simulink model "MSDRPrimaryLoop_LoadFollow"  (R2021b)
settings: Solver=VariableStepAuto  StartTime=0.0  StopTime=604900  MaxStep=1  MinStep=0.01  RelTol=1e-3
undefined symbols (not defined in the file): a_f, A_free_PHX, a_g, A_h_PHX, beta, beta_t, bubbleGeneratorArea, bubbleGeneratorDh, bubbleGeneratorElevation, bubbleGeneratorLength, bubbleGeneratorVolume, bubbleSaturationLevel, bubbleSeparatorArea, bubbleSeparatorDiameter, bubbleSeparatorDo, bubbleSeparatorLength, bubbleSeparatorSlope, bypassRatio, C0, coreFlowArea, coreFuelVolume, coreLowerPlenumArea, coreLowerPlenumHydraulicDiameter, coreLowerPlenumLength, coreLowerPlenumVolume, coreUpperPlenumArea, coreUpperPlenumHydraulicDiameter, coreUpperPlenumLength, coreUpperPlenumVolume, coreVolume, cpGraphite, dissolusionRatio, dMin, dScale, dsmConst, DXeG, Fiss_factor, fuelChannelHydrualicDiameter, fuelChannelLength, fuelDepositRatio, fuelFraction, fuelGraphiteArea, fuelGraphiteHeatTransferCoefficient, gamma0, gamma1, gamma2, generatorDsm, graphiteKDiff, graphiteUnitCellThickness, initialIodineConcentration, InitialXeMolarConcentration, InjectionRatio, injectionRatio, iodineDecayConstant, IodineDecayConstant, iodineYield, kGraphite, kScale, Lam, lam ... (+60)
libraries: fl_lib x268, nesl_utility x106, SimscapeFluids_lib x20, slpidlib x1
(part 3 of 12)

== system MSDRPrimaryLoop_LoadFollow/Pump/PumpPysical ==
  XeIn : Inport
  GasIn : Inport  Port=2
  Add : Sum  Inputs=|++
  Delay One Step : Delay  DelayLength=1
  Gain : Gain  Gain=0.5
  GasCalc : Subsystem
      settings: PortSchema="{\"entries\":[{\"content\":{\"sides\":[{\"content\":{\"connectorIds\":[\"In1\"]},\"type\":\"ConnectorPlacement.EquallySpacedRectSide\",\"uuid\":\"a8e1ce06-71c9-462d-8d5c-7a3e078b5544\"},{\"content\":{\"connectorIds\":[\"Out1\"],\"side\":\"RIGHT\"},\"type\":\"ConnectorPlacement.EquallySpacedRectSide\",\"uuid\":\"2c63a1ce-15e2-4b17-a432-f9f40781bd58\"},{\"content\":{\"connectorIds\":[\"LConn1\",\"LConn2\",\"LConn3\"],\"side\":\"TOP\"},\"type\":\"ConnectorPlacement.EquallySpacedRectSide\",\"uuid\":\"abc20e07-15eb-475f-be7f-cc96378523a1\"},{\"content\":{\"connectorIds\":[],\"side\":\"BOTTOM\"},\"type\":\"ConnectorPlacement.EquallySpacedRectSide\",\"uuid\":\"ab58f362-f4c2-4e86-bda0-802426066295\"}]},\"type\":\"ConnectorPlacement.EquallySpacedConnector\",\"uuid\":\"b54d49a9-048b-4912-bf18-92a7ef5e8aff\"}],\"packageUris\":[\"http://schema.mathworks.com/mf0/Connector/R2020b\"],\"version\":\"1.0\"}"
  PumpPhysics&Control : Subsystem
      settings: PortSchema="{\"entries\":[{\"content\":{\"sides\":[{\"content\":{\"connectorIds\":[\"LConn1\",\"In1\"]},\"type\":\"ConnectorPlacement.EquallySpacedRectSide\",\"uuid\":\"dfa2aa95-b0f6-4d42-b52c-ac64f68b4332\"},{\"content\":{\"connectorIds\":[\"RConn1\"],\"side\":\"RIGHT\"},\"type\":\"ConnectorPlacement.EquallySpacedRectSide\",\"uuid\":\"4e233f45-275b-4a62-b54f-a26261252d76\"},{\"content\":{\"connectorIds\":[],\"side\":\"TOP\"},\"type\":\"ConnectorPlacement.EquallySpacedRectSide\",\"uuid\":\"4d56cee6-54c9-4b53-b595-9dd9843d1812\"},{\"content\":{\"connectorIds\":[\"RConn2\"],\"side\":\"BOTTOM\"},\"type\":\"ConnectorPlacement.EquallySpacedRectSide\",\"uuid\":\"5b59abd0-5c01-4c9b-8b33-a5a665899d43\"}]},\"type\":\"ConnectorPlacement.EquallySpacedConnector\",\"uuid\":\"08118153-6206-4ac8-9187-5e3d4b128de1\"}],\"packageUris\":[\"http://schema.mathworks.com/mf0/Connector/R2020b\"],\"version\":\"1.0\"}"
  XenonCalc : Subsystem
      settings: PortSchema="{\"entries\":[{\"content\":{\"sides\":[{\"content\":{\"connectorIds\":[\"In1\"]},\"type\":\"ConnectorPlacement.EquallySpacedRectSide\",\"uuid\":\"2d0a178d-e3ce-4b60-98e7-1a8cc2d8e60a\"},{\"content\":{\"connectorIds\":[\"Out1\"],\"side\":\"RIGHT\"},\"type\":\"ConnectorPlacement.EquallySpacedRectSide\",\"uuid\":\"c836f1a2-1f60-4759-a54a-d13020949774\"},{\"content\":{\"connectorIds\":[\"LConn1\"],\"side\":\"TOP\"},\"type\":\"ConnectorPlacement.EquallySpacedRectSide\",\"uuid\":\"88d5b9ac-da0a-4ad3-844b-69cd646a8f29\"},{\"content\":{\"connectorIds\":[],\"side\":\"BOTTOM\"},\"type\":\"ConnectorPlacement.EquallySpacedRectSide\",\"uuid\":\"7af8c1ea-1928-402f-ba73-00fd41d484c9\"}]},\"type\":\"ConnectorPlacement.EquallySpacedConnector\",\"uuid\":\"10dc3dbd-7ee0-472f-a356-245132d02761\"}],\"packageUris\":[\"http://schema.mathworks.com/mf0/Connector/R2020b\"],\"version\":\"1.0\"}"
  Inlet : PMIOPort  Side=Left
  Outlet : PMIOPort  Port=2  Side=Right
  XeOut : Outport
  GasOut : Outport  Port=2
  wires:
  GasIn/1 -> GasCalc/1(GasIn), Add/1
  GasCalc/1(GasOut) -> GasOut/1, Add/2
  Add/1 -> Gain/1
  Gain/1 -> Delay One Step/1
  Delay One Step/1 -> PumpPhysics&Control/1(GasRef)
  XeIn/1 -> XenonCalc/1(XeIn)
  XenonCalc/1(XeOut) -> XeOut/1
  connections:
  Inlet/RConn1 -- GasCalc/LConn1 -- PumpPhysics&Control/LConn1
  Outlet/RConn1 -- PumpPhysics&Control/RConn1 -- GasCalc/LConn3
  PumpPhysics&Control/RConn2 -- GasCalc/LConn2 -- XenonCalc/LConn1

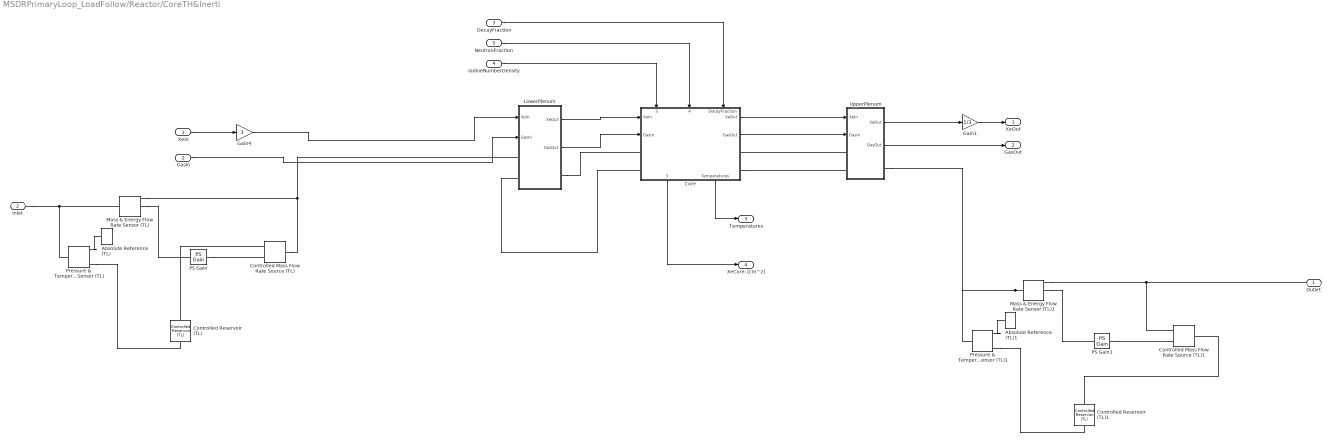
== system MSDRPrimaryLoop_LoadFollow/Reactor/CoreTH&Inerti ==
  XeIn : Inport
  GasIn : Inport  Port=2
  DecayFraction : Inport  Port=3
  IodineNumberDensity : Inport  Port=4
  NeutronFraction : Inport  Port=5
  Absolute Reference (TL) : fl_lib/Thermal Liquid/Elements/Absolute Reference (TL)
      settings: SourceProductBaseCode=SS
  Absolute Reference (TL)1 : fl_lib/Thermal Liquid/Elements/Absolute Reference (TL)
      settings: SourceProductBaseCode=SS
  Controlled Mass Flow Rate Source (TL) : fl_lib/Thermal Liquid/Sources/Controlled Mass Flow Rate Source (TL)  area=0.01 m^2
      settings: SourceProductBaseCode=SS  InternalSimscapePortConfiguration="{\"Bottom\":[],\"Left\":[{\"id\":\"A\",\"label\":\"A\",\"type\":\"foundation.thermal_liquid.thermal_liquid\"},{\"id\":\"M\",\"label\":\"M\",\"type\":\"input\"}],\"Right\":[{\"id\":\"B\",\"label\":\"B\",\"type\":\"foundation.thermal_liquid.thermal_liquid\"}],\"Top\":[]}"
  Controlled Mass Flow Rate Source (TL)1 : fl_lib/Thermal Liquid/Sources/Controlled Mass Flow Rate Source (TL)  area=0.01 m^2
      settings: SourceProductBaseCode=SS  InternalSimscapePortConfiguration="{\"Bottom\":[],\"Left\":[{\"id\":\"A\",\"label\":\"A\",\"type\":\"foundation.thermal_liquid.thermal_liquid\"},{\"id\":\"M\",\"label\":\"M\",\"type\":\"input\"}],\"Right\":[{\"id\":\"B\",\"label\":\"B\",\"type\":\"foundation.thermal_liquid.thermal_liquid\"}],\"Top\":[]}"
  Controlled Reservoir (TL) : fl_lib/Thermal Liquid/Elements/Controlled Reservoir (TL)  pressure_spec=foundation.enum.pressure_spec.atmospheric  reservoir_pressure=0.101325 MPa  area=0.01 m^2
      settings: SourceProductBaseCode=SS  InternalSimscapePortConfiguration="{\"Bottom\":[],\"Left\":[{\"id\":\"A\",\"label\":\"A\",\"type\":\"foundation.thermal_liquid.thermal_liquid\"}],\"Right\":[{\"id\":\"T_in\",\"label\":\"T\",\"type\":\"input\"}],\"Top\":[]}"
  Controlled Reservoir (TL)1 : fl_lib/Thermal Liquid/Elements/Controlled Reservoir (TL)  pressure_spec=foundation.enum.pressure_spec.atmospheric  reservoir_pressure=0.101325 MPa  area=0.01 m^2
      settings: SourceProductBaseCode=SS  InternalSimscapePortConfiguration="{\"Bottom\":[],\"Left\":[{\"id\":\"A\",\"label\":\"A\",\"type\":\"foundation.thermal_liquid.thermal_liquid\"}],\"Right\":[{\"id\":\"T_in\",\"label\":\"T\",\"type\":\"input\"}],\"Top\":[]}"
  Core : Subsystem
      settings: PortSchema="{\"entries\":[{\"content\":{\"sides\":[{\"content\":{\"connectorIds\":[\"In1\",\"In2\",\"LConn1\",\"LConn2\"]},\"type\":\"ConnectorPlacement.EquallySpacedRectSide\",\"uuid\":\"aa0e8e95-1a6b-4cbf-bd57-1ab05efc3e4b\"},{\"content\":{\"connectorIds\":[\"Out1\",\"Out2\",\"RConn1\",\"RConn2\"],\"side\":\"RIGHT\"},\"type\":\"ConnectorPlacement.EquallySpacedRectSide\",\"uuid\":\"e0eb6fcb-82a6-4aae-a4df-9b33aecd4e5c\"},{\"content\":{\"connectorIds\":[\"In3\",\"In4\",\"In5\"],\"side\":\"TOP\"},\"type\":\"ConnectorPlacement.EquallySpacedRectSide\",\"uuid\":\"5c074248-aee7-4f3a-b52e-673d2721cbd0\"},{\"content\":{\"connectorIds\":[\"Out3\",\"Out4\"],\"side\":\"BOTTOM\"},\"type\":\"ConnectorPlacement.EquallySpacedRectSide\",\"uuid\":\"89c6def1-6805-4ec7-892d-526461980e5e\"}]},\"type\":\"ConnectorPlacement.EquallySpacedConnector\",\"uuid\":\"cb503f6d-916e-44d8-aa57-58c36cce55e5\"}],\"packageUris\":[\"http://schema.mathworks.com/mf0/Connector/R2020b\"],\"version\":\"1.0\"}"
  Gain1 : Gain  Gain=1/3
  Gain4 : Gain  Gain=3
  LowerPlenum : Subsystem  mask{Volume=coreLowerPlenumVolume, Area=coreLowerPlenumArea, Length=coreLowerPlenumLength, Dh=coreLowerPlenumHydraulicDiameter, Elevation=coreLowerPlenumLength}
      mask prompts: Dh "Hydraulic Diameter"
  Mass & Energy Flow Rate Sensor (TL) : fl_lib/Thermal Liquid/Sensors/Mass & Energy Flow Rate Sensor (TL)
      settings: SourceProductBaseCode=SS  InternalSimscapePortConfiguration="{\"Bottom\":[],\"Left\":[{\"id\":\"A\",\"label\":\"A\",\"type\":\"foundation.thermal_liquid.thermal_liquid\"}],\"Right\":[{\"id\":\"B\",\"label\":\"B\",\"type\":\"foundation.thermal_liquid.thermal_liquid\"},{\"id\":\"M\",\"label\":\"M\",\"type\":\"output\"},{\"id\":\"PHI\",\"label\":\"Phi\",\"type\":\"output\"}],\"Top\":[]}"
  Mass & Energy Flow Rate Sensor (TL)1 : fl_lib/Thermal Liquid/Sensors/Mass & Energy Flow Rate Sensor (TL)
      settings: SourceProductBaseCode=SS  InternalSimscapePortConfiguration="{\"Bottom\":[],\"Left\":[{\"id\":\"A\",\"label\":\"A\",\"type\":\"foundation.thermal_liquid.thermal_liquid\"}],\"Right\":[{\"id\":\"B\",\"label\":\"B\",\"type\":\"foundation.thermal_liquid.thermal_liquid\"},{\"id\":\"M\",\"label\":\"M\",\"type\":\"output\"},{\"id\":\"PHI\",\"label\":\"Phi\",\"type\":\"output\"}],\"Top\":[]}"
  PS Gain : fl_lib/Physical Signals/Functions/PS Gain  gain=2
  PS Gain1 : fl_lib/Physical Signals/Functions/PS Gain  gain=2/3
  Pressure & Temperature Sensor (TL) : fl_lib/Thermal Liquid/Sensors/Pressure & Temperature Sensor (TL)
      settings: SourceProductBaseCode=SS  InternalSimscapePortConfiguration="{\"Bottom\":[],\"Left\":[{\"id\":\"A\",\"label\":\"A\",\"type\":\"foundation.thermal_liquid.thermal_liquid\"}],\"Right\":[{\"id\":\"B\",\"label\":\"B\",\"type\":\"foundation.thermal_liquid.thermal_liquid\"},{\"id\":\"P\",\"label\":\"P\",\"type\":\"output\"},{\"id\":\"T\",\"label\":\"T\",\"type\":\"output\"}],\"Top\":[]}"
  Pressure & Temperature Sensor (TL)1 : fl_lib/Thermal Liquid/Sensors/Pressure & Temperature Sensor (TL)
      settings: SourceProductBaseCode=SS  InternalSimscapePortConfiguration="{\"Bottom\":[],\"Left\":[{\"id\":\"A\",\"label\":\"A\",\"type\":\"foundation.thermal_liquid.thermal_liquid\"}],\"Right\":[{\"id\":\"B\",\"label\":\"B\",\"type\":\"foundation.thermal_liquid.thermal_liquid\"},{\"id\":\"P\",\"label\":\"P\",\"type\":\"output\"},{\"id\":\"T\",\"label\":\"T\",\"type\":\"output\"}],\"Top\":[]}"
  UpperPlenum : Subsystem  mask{Volume=coreUpperPlenumVolume, Area=coreUpperPlenumArea, Length=coreUpperPlenumLength, Dh=coreUpperPlenumHydraulicDiameter, Elevation=coreUpperPlenumLength}
      mask prompts: Dh "Hydraulic Diameter"
  Outlet : PMIOPort  Side=Right
  Inlet : PMIOPort  Port=2  Side=Left
  XeOut : Outport
  GasOut : Outport  Port=2
  Temperatures : Outport  Port=3
  "XeCore, [cm^2]" : Outport  Port=4
  wires:
  DecayFraction/1 -> Core/5(DecayFraction)
  NeutronFraction/1 -> Core/4(NeutronFraction)
  IodineNumberDensity/1 -> Core/3(IodineSNumberDensity)
  Core/3("TotalXeCrossSection, [cm^2]") -> "XeCore, [cm^2]"/1
  Core/4(Temperatures) -> Temperatures/1
  XeIn/1 -> Gain4/1
  Gain4/1 -> LowerPlenum/1(XeIn)
  GasIn/1 -> LowerPlenum/2(GasIn)
  LowerPlenum/1(XeOut) -> Core/1(XeIn)
  UpperPlenum/1(XeOut) -> Gain1/1
  Core/1(XeOut) -> UpperPlenum/1(XeIn)
  Core/2(GasOut) -> UpperPlenum/2(GasIn)
  LowerPlenum/2(GasOut) -> Core/2(GasIn)
  Gain1/1 -> XeOut/1
  UpperPlenum/2(GasOut) -> GasOut/1
  connections:
  LowerPlenum/LConn2 -- Core/LConn2
  Mass & Energy Flow Rate Sensor (TL)/RConn1 -- LowerPlenum/LConn1 -- Controlled Mass Flow Rate Source (TL)/RConn1
  LowerPlenum/RConn1 -- Core/LConn1
  UpperPlenum/LConn1 -- Core/RConn1
  Core/RConn2 -- UpperPlenum/LConn2
  Inlet/RConn1 -- Pressure & Temperature Sensor (TL)/LConn1 -- Mass & Energy Flow Rate Sensor (TL)/LConn1
  Pressure & Temperature Sensor (TL)/RConn1 -- Absolute Reference (TL)/LConn1
  Pressure & Temperature Sensor (TL)/RConn3 -- Controlled Reservoir (TL)/RConn1
  Controlled Reservoir (TL)/LConn1 -- Controlled Mass Flow Rate Source (TL)/LConn1
  Mass & Energy Flow Rate Sensor (TL)/RConn2 -- PS Gain/LConn1
  PS Gain/RConn1 -- Controlled Mass Flow Rate Source (TL)/LConn2
  Mass & Energy Flow Rate Sensor (TL)1/LConn1 -- UpperPlenum/RConn1 -- Pressure & Temperature Sensor (TL)1/LConn1
  Mass & Energy Flow Rate Sensor (TL)1/RConn1 -- Controlled Mass Flow Rate Source (TL)1/LConn1 -- Outlet/RConn1
  PS Gain1/RConn1 -- Controlled Mass Flow Rate Source (TL)1/LConn2
  Mass & Energy Flow Rate Sensor (TL)1/RConn2 -- PS Gain1/LConn1
  Pressure & Temperature Sensor (TL)1/RConn3 -- Controlled Reservoir (TL)1/RConn1
  Pressure & Temperature Sensor (TL)1/RConn1 -- Absolute Reference (TL)1/LConn1
  Controlled Reservoir (TL)1/LConn1 -- Controlled Mass Flow Rate Source (TL)1/RConn1

== system MSDRPrimaryLoop_LoadFollow/Reactor/Decay Heat ==
  note: Reference from UTK MSDR model
  (n/n_0) : Inport
  Decay Power Percentage : Fcn  Expr=u(2)+u(3)+u(4)
  Decay Precursor G1 : Fcn  Expr=u(1)*Fiss_factor*gamma0 - lambda0*u(2)
  Decay Precursor G2 : Fcn  Expr=u(1)*Fiss_factor*gamma1 - lambda1*u(3)
  Decay Precursor G3 : Fcn  Expr=u(1)*Fiss_factor*gamma2 - lambda2*u(4)
  Integrator : Integrator  InitialCondition=0.025125
  Integrator1 : Integrator  InitialCondition=0.0198578
  Integrator2 : Integrator  InitialCondition=0.0227606
  Mux : Mux
      settings: DisplayOption=signals
  "Relative Decay Power " : Outport  VectorParamsAs1DForOutWhenUnconnected=off
  wires:
  Decay Power Percentage/1 -> "Relative Decay Power "/1
  Decay Precursor G1/1 -> Integrator/1
  Decay Precursor G2/1 -> Integrator1/1
  Decay Precursor G3/1 -> Integrator2/1
  Mux/1 -> Decay Precursor G3/1, Decay Precursor G2/1, Decay Precursor G1/1, Decay Power Percentage/1
  Integrator/1 -> Mux/2
  Integrator1/1 -> Mux/3
  Integrator2/1 -> Mux/4
  (n/n_0)/1 -> Mux/1

== system MSDRPrimaryLoop_LoadFollow/Reactor/FlowFraction ==
  PS Abs : fl_lib/Physical Signals/Nonlinear Operators/PS Abs
      settings: SourceProductBaseCode=SS  InternalSimscapePortConfiguration="{\"Bottom\":[],\"Left\":[{\"id\":\"I\",\"label\":\"\",\"type\":\"input\"}],\"Right\":[{\"id\":\"O\",\"label\":\"\",\"type\":\"output\"}],\"Top\":[]}"
  PS Constant : fl_lib/Physical Signals/Sources/PS Constant  constant=nominalDischargeRate m^3/s
  PS Constant1 : fl_lib/Physical Signals/Sources/PS Constant  constant=0.1
  PS Divide : fl_lib/Physical Signals/Functions/PS Divide
      settings: SourceProductBaseCode=SS
  PS Max : fl_lib/Physical Signals/Nonlinear Operators/PS Max
      settings: SourceProductBaseCode=SS  InternalSimscapePortConfiguration="{\"Bottom\":[],\"Left\":[{\"id\":\"I1\",\"label\":\"\",\"type\":\"input\"},{\"id\":\"I2\",\"label\":\"\",\"type\":\"input\"}],\"Right\":[{\"id\":\"O\",\"label\":\"\",\"type\":\"output\"}],\"Top\":[]}"
  PS-Simulink Converter : nesl_utility/PS-Simulink Converter  PhysicalDomain=network_engine_domain  SubClassName=ps_output  LeftPortType=input  RightPortType=output  PseudoPeriodic=off  Frequencies=[]  Unit=inherit  AffineConversion=off
      settings: SourceProductBaseCode=PW,SS
  Volumetric Flow Rate Sensor (TL) : fl_lib/Thermal Liquid/Sensors/Volumetric Flow Rate Sensor (TL)
      settings: SourceProductBaseCode=SS  InternalSimscapePortConfiguration="{\"Bottom\":[],\"Left\":[{\"id\":\"A\",\"label\":\"A\",\"type\":\"foundation.thermal_liquid.thermal_liquid\"}],\"Right\":[{\"id\":\"B\",\"label\":\"B\",\"type\":\"foundation.thermal_liquid.thermal_liquid\"},{\"id\":\"V\",\"label\":\"V\",\"type\":\"output\"}],\"Top\":[]}"
  Outlet : PMIOPort  Side=Left
  Inlet : PMIOPort  Port=2  Side=Right
  FlowFrac : Outport
  wires:
  PS-Simulink Converter/1 -> FlowFrac/1
  connections:
  Inlet/RConn1 -- Volumetric Flow Rate Sensor (TL)/LConn1
  PS Divide/RConn1 -- PS Max/LConn1
  PS Abs/LConn1 -- Volumetric Flow Rate Sensor (TL)/RConn2
  PS Abs/RConn1 -- PS Divide/LConn1
  Volumetric Flow Rate Sensor (TL)/RConn1 -- Outlet/RConn1
  PS Constant/RConn1 -- PS Divide/LConn2
  PS Constant1/RConn1 -- PS Max/LConn2
  PS-Simulink Converter/LConn1 -- PS Max/RConn1

== system MSDRPrimaryLoop_LoadFollow/Reactor/Iodine ==
  NeutronFraction : Inport
  IodineAtoms : Integrator  InitialCondition=nominalFissionRate*iodineYield/iodineDecayConstant*initialIodineConcentration
  IodineDecay : Gain  Gain=iodineDecayConstant
  "IodineGeneration, [1/s]" : Product
  IodineYield : Constant  Value=iodineYield
  NominalFissionRate : Constant  Value=nominalFissionRate
  Product : Product
  Sum : Sum  Inputs=|+-
  TotalFuelMass : Gain  Gain=1/TotalFuelMass
  IodineSpecificNumberDensity : Outport
  wires:
  NeutronFraction/1 -> Product/1
  NominalFissionRate/1 -> Product/2
  Product/1 -> "IodineGeneration, [1/s]"/1
  IodineYield/1 -> "IodineGeneration, [1/s]"/2
  "IodineGeneration, [1/s]"/1 -> Sum/1
  Sum/1 -> IodineAtoms/1
  IodineAtoms/1 -> TotalFuelMass/1, IodineDecay/1
  IodineDecay/1 -> Sum/2
  TotalFuelMass/1 -> IodineSpecificNumberDensity/1

== system MSDRPrimaryLoop_LoadFollow/Reactor/Reactivity&PKE ==
  "XeCore, [cm^2]" : Inport
  FlowFrac : Inport  Port=2
  CORE TEMPERATURE : Inport  Port=3
  Ideal : Subsystem  Tag=Ideal  VariantControl=Ideal
      settings: PortSchema="{\"entries\":[{\"content\":{\"sides\":[{\"content\":{\"connectorIds\":[\"In1\",\"In2\"]},\"type\":\"ConnectorPlacement.EquallySpacedRectSide\",\"uuid\":\"074f11f6-c1de-4c2b-8a0d-6fb79ace2562\"},{\"content\":{\"connectorIds\":[\"Out1\"],\"side\":\"RIGHT\"},\"type\":\"ConnectorPlacement.EquallySpacedRectSide\",\"uuid\":\"1e53023e-28a9-4bb2-a66a-dc8b20408ca8\"},{\"content\":{\"connectorIds\":[\"In3\"],\"side\":\"TOP\"},\"type\":\"ConnectorPlacement.EquallySpacedRectSide\",\"uuid\":\"c85bb8ca-746f-4c14-b3fb-421abac5a8d5\"}]},\"type\":\"ConnectorPlacement.EquallySpacedConnector\",\"uuid\":\"7a35571e-b06b-4c7c-9209-bb340882391c\"}],\"packageUris\":[\"http://schema.mathworks.com/mf0/Connector/R2020b\"],\"version\":\"1.0\"}"
  Reactivity&PKE : Subsystem  Tag=PKE  VariantControl=PKE
      settings: PortSchema="{\"entries\":[{\"content\":{\"sides\":[{\"content\":{\"connectorIds\":[\"In1\",\"In2\"]},\"type\":\"ConnectorPlacement.EquallySpacedRectSide\",\"uuid\":\"074f11f6-c1de-4c2b-8a0d-6fb79ace2562\"},{\"content\":{\"connectorIds\":[\"Out1\"],\"side\":\"RIGHT\"},\"type\":\"ConnectorPlacement.EquallySpacedRectSide\",\"uuid\":\"1e53023e-28a9-4bb2-a66a-dc8b20408ca8\"},{\"content\":{\"connectorIds\":[],\"side\":\"TOP\"},\"type\":\"ConnectorPlacement.EquallySpacedRectSide\",\"uuid\":\"c85bb8ca-746f-4c14-b3fb-421abac5a8d5\"},{\"content\":{\"connectorIds\":[\"In3\"],\"side\":\"BOTTOM\"},\"type\":\"ConnectorPlacement.EquallySpacedRectSide\",\"uuid\":\"b54f140c-bd85-4d1d-bf3e-e1de5989b678\"}]},\"type\":\"ConnectorPlacement.EquallySpacedConnector\",\"uuid\":\"7a35571e-b06b-4c7c-9209-bb340882391c\"}],\"packageUris\":[\"http://schema.mathworks.com/mf0/Connector/R2020b\"],\"version\":\"1.0\"}"
  FRACTIONAL NEUTRON DENSITY : Outport

== system MSDRPrimaryLoop_LoadFollow/pipePHXToReactor/GasCalc ==
  GasIn : Inport
  Add : Sum  Inputs=+-
  GasExpansion : Subsystem  ReferencedSubsystem=GasExpansion
      settings: PortSchema="{\"entries\":[{\"content\":{\"sides\":[{\"content\":{\"connectorIds\":[\"LConn1\",\"In1\"]},\"type\":\"ConnectorPlacement.EquallySpacedRectSide\",\"uuid\":\"50c89675-cb8a-4964-af62-cb2014507b1d\"},{\"content\":{\"connectorIds\":[\"RConn1\",\"Out1\"],\"side\":\"RIGHT\"},\"type\":\"ConnectorPlacement.EquallySpacedRectSide\",\"uuid\":\"6b3adc78-0be5-4682-9da0-6fd41ffc4e71\"},{\"content\":{\"connectorIds\":[],\"side\":\"TOP\"},\"type\":\"ConnectorPlacement.EquallySpacedRectSide\",\"uuid\":\"5158b46f-a496-48e4-90d6-6c6dcc9e237b\"}]},\"type\":\"ConnectorPlacement.EquallySpacedConnector\",\"uuid\":\"7ff0188e-dc19-44a0-a8cf-bde33949414f\"}],\"packageUris\":[\"http://schema.mathworks.com/mf0/Connector/R2020b\"],\"version\":\"1.0\"}"
  Integrator : Integrator
  PS-Simulink Converter : nesl_utility/PS-Simulink Converter  PhysicalDomain=network_engine_domain  SubClassName=ps_output  LeftPortType=input  RightPortType=output  PseudoPeriodic=off  Frequencies=[]  Unit=inherit  AffineConversion=off
      settings: SourceProductBaseCode=PW,SS
  Product : Product
  VolumeToVoid : Gain  Gain=1/Volume
  Ref1 : PMIOPort  Side=Left
  VolumeRate : PMIOPort  Port=2  Side=Left
  Ref2 : PMIOPort  Port=3  Side=Left
  GasOut : Outport
  wires:
  VolumeToVoid/1 -> GasExpansion/1, Add/2
  Integrator/1 -> VolumeToVoid/1
  GasIn/1 -> Add/1
  Add/1 -> Product/1
  Product/1 -> Integrator/1
  PS-Simulink Converter/1 -> Product/2
  GasExpansion/1 -> GasOut/1
  connections:
  PS-Simulink Converter/LConn1 -- VolumeRate/RConn1
  GasExpansion/LConn1 -- Ref1/RConn1
  GasExpansion/RConn1 -- Ref2/RConn1

== system MSDRPrimaryLoop_LoadFollow/pipePHXToReactor/PLossFunc ==
  Constant : Constant  Value=Elevation*9.82
  PS-Simulink Converter : nesl_utility/PS-Simulink Converter  PhysicalDomain=network_engine_domain  SubClassName=ps_output  LeftPortType=input  RightPortType=output  PseudoPeriodic=off  Frequencies=[]  Unit=inherit  AffineConversion=off
      settings: SourceProductBaseCode=PW,SS
  PS-Simulink Converter1 : nesl_utility/PS-Simulink Converter  PhysicalDomain=network_engine_domain  SubClassName=ps_output  LeftPortType=input  RightPortType=output  PseudoPeriodic=off  Frequencies=[]  Unit=inherit  AffineConversion=off
      settings: SourceProductBaseCode=PW,SS
  Pressure & Temperature Sensor (TL) : fl_lib/Thermal Liquid/Sensors/Pressure & Temperature Sensor (TL)
      settings: SourceProductBaseCode=SS  InternalSimscapePortConfiguration="{\"Bottom\":[],\"Left\":[{\"id\":\"A\",\"label\":\"A\",\"type\":\"foundation.thermal_liquid.thermal_liquid\"}],\"Right\":[{\"id\":\"B\",\"label\":\"B\",\"type\":\"foundation.thermal_liquid.thermal_liquid\"},{\"id\":\"P\",\"label\":\"P\",\"type\":\"output\"},{\"id\":\"T\",\"label\":\"T\",\"type\":\"output\"}],\"Top\":[]}"
  Product : Product
  Subtract : Sum  Inputs=+-
  Thermodynamic Properties Sensor (TL) : fl_lib/Thermal Liquid/Sensors/Thermodynamic Properties Sensor (TL)
      settings: SourceProductBaseCode=SS  InternalSimscapePortConfiguration="{\"Bottom\":[],\"Left\":[{\"id\":\"A\",\"label\":\"A\",\"type\":\"foundation.thermal_liquid.thermal_liquid\"}],\"Right\":[{\"id\":\"U\",\"label\":\"u\",\"type\":\"output\"},{\"id\":\"RHO\",\"label\":\"rho\",\"type\":\"output\"},{\"id\":\"CP\",\"label\":\"cp\",\"type\":\"output\"}],\"Top\":[]}"
  Ref1 : PMIOPort  Side=Left
  Ref2 : PMIOPort  Port=2  Side=Right
  PLoss : Outport
  wires:
  PS-Simulink Converter1/1 -> Product/1
  PS-Simulink Converter/1 -> Subtract/1
  Product/1 -> Subtract/2
  Constant/1 -> Product/2
  Subtract/1 -> PLoss/1
  connections:
  Thermodynamic Properties Sensor (TL)/LConn1 -- Pressure & Temperature Sensor (TL)/RConn1 -- Ref2/RConn1
  PS-Simulink Converter/LConn1 -- Pressure & Temperature Sensor (TL)/RConn2
  Thermodynamic Properties Sensor (TL)/RConn2 -- PS-Simulink Converter1/LConn1
  Pressure & Temperature Sensor (TL)/LConn1 -- Ref1/RConn1

== system MSDRPrimaryLoop_LoadFollow/pipePHXToReactor/Subsystem ==
  note: Dh
  note: Dh
  note: Dh
  GasInRef : Inport
  2PModification : Subsystem  ReferencedSubsystem=TwoPhaseModification
      settings: PortSchema="{\"entries\":[{\"content\":{\"sides\":[{\"content\":{\"connectorIds\":[\"LConn1\"]},\"type\":\"ConnectorPlacement.EquallySpacedRectSide\",\"uuid\":\"7546b4b7-b669-49c8-8f27-f696391ea3ad\"},{\"content\":{\"connectorIds\":[\"RConn1\"],\"side\":\"RIGHT\"},\"type\":\"ConnectorPlacement.EquallySpacedRectSide\",\"uuid\":\"0e6176f2-177c-4327-bcfa-9a190fe9083f\"},{\"content\":{\"connectorIds\":[\"LConn2\"],\"side\":\"TOP\"},\"type\":\"ConnectorPlacement.EquallySpacedRectSide\",\"uuid\":\"16faf74c-4635-4009-a5b3-33dd03b625c6\"},{\"content\":{\"connectorIds\":[\"RConn2\",\"In1\"],\"side\":\"BOTTOM\"},\"type\":\"ConnectorPlacement.EquallySpacedRectSide\",\"uuid\":\"2081d73b-bb08-4ad9-b5c8-e48a4e9c4e20\"}]},\"type\":\"ConnectorPlacement.EquallySpacedConnector\",\"uuid\":\"243e4075-206b-4747-a8bc-b8f10d9a577f\"}],\"packageUris\":[\"http://schema.mathworks.com/mf0/Connector/R2020b\"],\"version\":\"1.0\"}"
  PS Abs : fl_lib/Physical Signals/Nonlinear Operators/PS Abs
      settings: SourceProductBaseCode=SS  InternalSimscapePortConfiguration="{\"Bottom\":[],\"Left\":[{\"id\":\"I\",\"label\":\"\",\"type\":\"input\"}],\"Right\":[{\"id\":\"O\",\"label\":\"\",\"type\":\"output\"}],\"Top\":[]}"
  Pipe (TL) : SimscapeFluids_lib/Thermal Liquid/Pipes & Fittings/Pipe (TL)  dynamic_compressibility=simscape.enum.onoff.on  inertia=simscape.enum.onoff.on  num_segments=1  pipe_length=Length m  area=Area m^2  Dh=0.1128 m  wall_spec=fluids.thermal_liquid.pipes_fittings.enum.wall_spec.rigid  Dh_rigid=Dh m  wall_compliance=1.2e-6 m/MPa  wall_time_constant=0.01 s  elevation_spec=foundation.enum.constant_variable.constant  elevation_gain=Elevation m  g=9.82 m/s^2  pressure_loss_spec=fluids.thermal_liquid.pipes_fittings.enum.PressureLossSpec.Haaland  length_add=1 m  roughness=15e-6 m  Re_friction_TLU=[400, 1000, 1500, 3000, 4000, 6000, 10000, 20000, 40000, 60000, 100000, 100000000]  friction_factor_TLU=[.264, .112, .071, .0417, .0387, .0268, .025, .0232, .0226, .022, .0214, .0214]  shape_factor=64  Re_lam=2000  Re_tur=4000  mdot_nominal=[.1, 1] kg/s  p_diff_nominal=[.001, .01] MPa  mdot_threshold=1e-6 kg/s  heat_transfer_spec=fluids.thermal_liquid.pipes_fittings.enum.HeatTransferSpec.Gnielinski  mdot_nominal_heat=[.1, 1] kg/s  T_in_nominal=[293.15, 293.15] K  T_out_nominal=[300, 300] K  p_in_nominal_heat=[.101325, .101325] MPa  T_wall_nominal=[303.15, 303.15] K  a_coeff=0.023  b_Re_power=0.8  c_Pr_power=0.4  Nu_lam=3.66  Re_Colburn_TLU=[100, 150, 1000]  Colburn_factor_TLU=[.019, .013, .002]  Re_Nu_TLU=[100, 150, 1000]  Pr_Nu_TLU=[1, 10]  Nu_TLU=[3.72, 4.21; 3.75, 4.44; 4.21, 7.15]  T0_vec=T0 K  p0_vec=P0 Pa  mdot0=0.1 kg/s
      settings: SourceProductBaseCode=SH  LogSimulationData=on
  Volumetric Flow Rate Sensor (TL) : fl_lib/Thermal Liquid/Sensors/Volumetric Flow Rate Sensor (TL)
      settings: SourceProductBaseCode=SS  InternalSimscapePortConfiguration="{\"Bottom\":[],\"Left\":[{\"id\":\"A\",\"label\":\"A\",\"type\":\"foundation.thermal_liquid.thermal_liquid\"}],\"Right\":[{\"id\":\"B\",\"label\":\"B\",\"type\":\"foundation.thermal_liquid.thermal_liquid\"},{\"id\":\"V\",\"label\":\"V\",\"type\":\"output\"}],\"Top\":[]}"
  Inlet : PMIOPort  Side=Left
  Outlet : PMIOPort  Port=2  Side=Right
  VolumeRate : PMIOPort  Port=3  Side=Right
  wires:
  GasInRef/1 -> 2PModification/1
  connections:
  Volumetric Flow Rate Sensor (TL)/RConn1 -- Pipe (TL)/LConn1
  Inlet/RConn1 -- 2PModification/LConn2 -- Volumetric Flow Rate Sensor (TL)/LConn1
  Pipe (TL)/RConn1 -- 2PModification/RConn2 -- 2PModification/LConn1
  Volumetric Flow Rate Sensor (TL)/RConn2 -- PS Abs/LConn1
  PS Abs/RConn1 -- VolumeRate/RConn1
  2PModification/RConn1 -- Outlet/RConn1

== system MSDRPrimaryLoop_LoadFollow/pipePHXToReactor/XenonCalc ==
  XeIn : Inport  OutDataTypeStr=double  Unit=kg/s
  PLoss : Inport  Port=2
  GasRef : Inport  Port=3
  Absolute Reference (TL) : fl_lib/Thermal Liquid/Elements/Absolute Reference (TL)
      settings: SourceProductBaseCode=SS
  Demux : Demux  Outputs=2
  Gas : Subsystem
      settings: PortSchema="{\"entries\":[{\"content\":{\"sides\":[{\"content\":{\"connectorIds\":[\"In1\"]},\"type\":\"ConnectorPlacement.EquallySpacedRectSide\",\"uuid\":\"9457d014-8c8c-4ede-953a-dad1b8fcff2e\"},{\"content\":{\"connectorIds\":[\"Out1\"],\"side\":\"RIGHT\"},\"type\":\"ConnectorPlacement.EquallySpacedRectSide\",\"uuid\":\"6b13e550-1648-4662-a58b-f6f49b8dfc45\"},{\"content\":{\"connectorIds\":[\"Out2\",\"In2\"],\"side\":\"TOP\"},\"type\":\"ConnectorPlacement.EquallySpacedRectSide\",\"uuid\":\"73a4211d-b4c2-4f72-9c26-6ee46c1777bd\"},{\"content\":{\"connectorIds\":[\"In3\",\"In4\"],\"side\":\"BOTTOM\"},\"type\":\"ConnectorPlacement.EquallySpacedRectSide\",\"uuid\":\"ca62b0cd-46c8-418f-9a8b-9558726bf444\"}]},\"type\":\"ConnectorPlacement.EquallySpacedConnector\",\"uuid\":\"020f2da1-56fe-4a8a-8a2d-2f75d9123e14\"}],\"packageUris\":[\"http://schema.mathworks.com/mf0/Connector/R2020b\"],\"version\":\"1.0\"}"
  InterphaseTranfser : Subsystem
      settings: PortSchema="{\"entries\":[{\"content\":{\"sides\":[{\"content\":{\"connectorIds\":[\"In1\",\"In2\",\"In3\"]},\"type\":\"ConnectorPlacement.EquallySpacedRectSide\",\"uuid\":\"d6303689-138e-451a-a3c3-60d601b4795c\"},{\"content\":{\"connectorIds\":[\"In5\",\"Out1\"],\"side\":\"RIGHT\"},\"type\":\"ConnectorPlacement.EquallySpacedRectSide\",\"uuid\":\"e99266db-1ad9-4248-a3a9-dc80edd4cbf2\"},{\"content\":{\"connectorIds\":[\"LConn1\"],\"side\":\"TOP\"},\"type\":\"ConnectorPlacement.EquallySpacedRectSide\",\"uuid\":\"07679a3e-e535-452f-8d16-cac9376cf8bb\"},{\"content\":{\"connectorIds\":[\"In4\"],\"side\":\"BOTTOM\"},\"type\":\"ConnectorPlacement.EquallySpacedRectSide\",\"uuid\":\"cd334689-6a33-4cbf-8721-40055306f60f\"}]},\"type\":\"ConnectorPlacement.EquallySpacedConnector\",\"uuid\":\"2a8870ca-366d-4312-85a0-e0a2095078d0\"}],\"packageUris\":[\"http://schema.mathworks.com/mf0/Connector/R2020b\"],\"version\":\"1.0\"}"
  Mux : Mux  Inputs=2
  PS Abs : fl_lib/Physical Signals/Nonlinear Operators/PS Abs
      settings: SourceProductBaseCode=SS  InternalSimscapePortConfiguration="{\"Bottom\":[],\"Left\":[{\"id\":\"I\",\"label\":\"\",\"type\":\"input\"}],\"Right\":[{\"id\":\"O\",\"label\":\"\",\"type\":\"output\"}],\"Top\":[]}"
  PS-Simulink Converter : nesl_utility/PS-Simulink Converter  PhysicalDomain=network_engine_domain  SubClassName=ps_output  LeftPortType=input  RightPortType=output  PseudoPeriodic=off  Frequencies=[]  Unit=inherit  AffineConversion=off
      settings: SourceProductBaseCode=PW,SS
  PS-Simulink Converter1 : nesl_utility/PS-Simulink Converter  PhysicalDomain=network_engine_domain  SubClassName=ps_output  LeftPortType=input  RightPortType=output  PseudoPeriodic=off  Frequencies=[]  Unit=inherit  AffineConversion=off
      settings: SourceProductBaseCode=PW,SS
  Pressure & Temperature Sensor (TL) : fl_lib/Thermal Liquid/Sensors/Pressure & Temperature Sensor (TL)
      settings: SourceProductBaseCode=SS  InternalSimscapePortConfiguration="{\"Bottom\":[],\"Left\":[{\"id\":\"A\",\"label\":\"A\",\"type\":\"foundation.thermal_liquid.thermal_liquid\"}],\"Right\":[{\"id\":\"B\",\"label\":\"B\",\"type\":\"foundation.thermal_liquid.thermal_liquid\"},{\"id\":\"P\",\"label\":\"P\",\"type\":\"output\"},{\"id\":\"T\",\"label\":\"T\",\"type\":\"output\"}],\"Top\":[]}"
  Salt : Subsystem
      settings: PortSchema="{\"entries\":[{\"content\":{\"sides\":[{\"content\":{\"connectorIds\":[\"In1\",\"In2\",\"In3\"]},\"type\":\"ConnectorPlacement.EquallySpacedRectSide\",\"uuid\":\"9457d014-8c8c-4ede-953a-dad1b8fcff2e\"},{\"content\":{\"connectorIds\":[\"Out1\"],\"side\":\"RIGHT\"},\"type\":\"ConnectorPlacement.EquallySpacedRectSide\",\"uuid\":\"6b13e550-1648-4662-a58b-f6f49b8dfc45\"},{\"content\":{\"connectorIds\":[\"In4\",\"In5\"],\"side\":\"TOP\"},\"type\":\"ConnectorPlacement.EquallySpacedRectSide\",\"uuid\":\"73a4211d-b4c2-4f72-9c26-6ee46c1777bd\"},{\"content\":{\"connectorIds\":[\"Out2\",\"In6\"],\"side\":\"BOTTOM\"},\"type\":\"ConnectorPlacement.EquallySpacedRectSide\",\"uuid\":\"ca62b0cd-46c8-418f-9a8b-9558726bf444\"}]},\"type\":\"ConnectorPlacement.EquallySpacedConnector\",\"uuid\":\"020f2da1-56fe-4a8a-8a2d-2f75d9123e14\"}],\"packageUris\":[\"http://schema.mathworks.com/mf0/Connector/R2020b\"],\"version\":\"1.0\"}"
  Volumetric Flow Rate Sensor (TL) : fl_lib/Thermal Liquid/Sensors/Volumetric Flow Rate Sensor (TL)
      settings: SourceProductBaseCode=SS  InternalSimscapePortConfiguration="{\"Bottom\":[],\"Left\":[{\"id\":\"A\",\"label\":\"A\",\"type\":\"foundation.thermal_liquid.thermal_liquid\"}],\"Right\":[{\"id\":\"B\",\"label\":\"B\",\"type\":\"foundation.thermal_liquid.thermal_liquid\"},{\"id\":\"V\",\"label\":\"V\",\"type\":\"output\"}],\"Top\":[]}"
  Inlet : PMIOPort  Side=Left
  Outlet : PMIOPort  Port=2  Side=Right
  XeOut : Outport
  wires:
  XeIn/1 -> Demux/1
  PS-Simulink Converter/1 -> InterphaseTranfser/5(VolumeRate), Gas/4(VolumeRate), Salt/5(VolumeRate)
  GasRef/1 -> Gas/3(GasRef), InterphaseTranfser/2(GasRef), Salt/4(GasRef)
  Demux/1 -> Salt/1(XeLIn)
  [IodineSNDensity] -> Salt/2(IodineSNumberDensity)
  Demux/2 -> Gas/1(XeGIn)
  Salt/1(XeLOut) -> Mux/1
  Gas/1(XeGOut) -> Mux/2
  Mux/1 -> XeOut/1
  Salt/2(GxSalt) -> InterphaseTranfser/1(GxSalt)
  Gas/2(GxGas) -> InterphaseTranfser/3(GxGas)
  InterphaseTranfser/1(TranfserRate) -> Salt/6(Interphase), Gas/2(Interphase)
  PS-Simulink Converter1/1 -> Salt/3(T_f_ave)
  PLoss/1 -> InterphaseTranfser/4(PLoss)
  connections:
  Outlet/RConn1 -- Volumetric Flow Rate Sensor (TL)/RConn1 -- InterphaseTranfser/LConn1
  Volumetric Flow Rate Sensor (TL)/LConn1 -- Pressure & Temperature Sensor (TL)/LConn1 -- Inlet/RConn1
  Volumetric Flow Rate Sensor (TL)/RConn2 -- PS Abs/LConn1
  PS Abs/RConn1 -- PS-Simulink Converter/LConn1
  Pressure & Temperature Sensor (TL)/RConn1 -- Absolute Reference (TL)/LConn1
  Pressure & Temperature Sensor (TL)/RConn3 -- PS-Simulink Converter1/LConn1

== system MSDRPrimaryLoop_LoadFollow/pipePumpToPHX/GasCalc ==
  GasIn : Inport
  Add : Sum  Inputs=+-
  GasExpansion : Subsystem  ReferencedSubsystem=GasExpansion
      settings: PortSchema="{\"entries\":[{\"content\":{\"sides\":[{\"content\":{\"connectorIds\":[\"LConn1\",\"In1\"]},\"type\":\"ConnectorPlacement.EquallySpacedRectSide\",\"uuid\":\"50c89675-cb8a-4964-af62-cb2014507b1d\"},{\"content\":{\"connectorIds\":[\"RConn1\",\"Out1\"],\"side\":\"RIGHT\"},\"type\":\"ConnectorPlacement.EquallySpacedRectSide\",\"uuid\":\"6b3adc78-0be5-4682-9da0-6fd41ffc4e71\"},{\"content\":{\"connectorIds\":[],\"side\":\"TOP\"},\"type\":\"ConnectorPlacement.EquallySpacedRectSide\",\"uuid\":\"5158b46f-a496-48e4-90d6-6c6dcc9e237b\"}]},\"type\":\"ConnectorPlacement.EquallySpacedConnector\",\"uuid\":\"7ff0188e-dc19-44a0-a8cf-bde33949414f\"}],\"packageUris\":[\"http://schema.mathworks.com/mf0/Connector/R2020b\"],\"version\":\"1.0\"}"
  Integrator : Integrator
  PS-Simulink Converter : nesl_utility/PS-Simulink Converter  PhysicalDomain=network_engine_domain  SubClassName=ps_output  LeftPortType=input  RightPortType=output  PseudoPeriodic=off  Frequencies=[]  Unit=inherit  AffineConversion=off
      settings: SourceProductBaseCode=PW,SS
  Product : Product
  VolumeToVoid : Gain  Gain=1/Volume
  Ref1 : PMIOPort  Side=Left
  VolumeRate : PMIOPort  Port=2  Side=Left
  Ref2 : PMIOPort  Port=3  Side=Left
  GasOut : Outport
  wires:
  VolumeToVoid/1 -> GasExpansion/1, Add/2
  Integrator/1 -> VolumeToVoid/1
  GasIn/1 -> Add/1
  Add/1 -> Product/1
  Product/1 -> Integrator/1
  PS-Simulink Converter/1 -> Product/2
  GasExpansion/1 -> GasOut/1
  connections:
  PS-Simulink Converter/LConn1 -- VolumeRate/RConn1
  GasExpansion/LConn1 -- Ref1/RConn1
  GasExpansion/RConn1 -- Ref2/RConn1

== system MSDRPrimaryLoop_LoadFollow/pipePumpToPHX/PLossFunc ==
  Constant : Constant  Value=Elevation*9.82
  PS-Simulink Converter : nesl_utility/PS-Simulink Converter  PhysicalDomain=network_engine_domain  SubClassName=ps_output  LeftPortType=input  RightPortType=output  PseudoPeriodic=off  Frequencies=[]  Unit=inherit  AffineConversion=off
      settings: SourceProductBaseCode=PW,SS
  PS-Simulink Converter1 : nesl_utility/PS-Simulink Converter  PhysicalDomain=network_engine_domain  SubClassName=ps_output  LeftPortType=input  RightPortType=output  PseudoPeriodic=off  Frequencies=[]  Unit=inherit  AffineConversion=off
      settings: SourceProductBaseCode=PW,SS
  Pressure & Temperature Sensor (TL) : fl_lib/Thermal Liquid/Sensors/Pressure & Temperature Sensor (TL)
      settings: SourceProductBaseCode=SS  InternalSimscapePortConfiguration="{\"Bottom\":[],\"Left\":[{\"id\":\"A\",\"label\":\"A\",\"type\":\"foundation.thermal_liquid.thermal_liquid\"}],\"Right\":[{\"id\":\"B\",\"label\":\"B\",\"type\":\"foundation.thermal_liquid.thermal_liquid\"},{\"id\":\"P\",\"label\":\"P\",\"type\":\"output\"},{\"id\":\"T\",\"label\":\"T\",\"type\":\"output\"}],\"Top\":[]}"
  Product : Product
  Subtract : Sum  Inputs=+-
  Thermodynamic Properties Sensor (TL) : fl_lib/Thermal Liquid/Sensors/Thermodynamic Properties Sensor (TL)
      settings: SourceProductBaseCode=SS  InternalSimscapePortConfiguration="{\"Bottom\":[],\"Left\":[{\"id\":\"A\",\"label\":\"A\",\"type\":\"foundation.thermal_liquid.thermal_liquid\"}],\"Right\":[{\"id\":\"U\",\"label\":\"u\",\"type\":\"output\"},{\"id\":\"RHO\",\"label\":\"rho\",\"type\":\"output\"},{\"id\":\"CP\",\"label\":\"cp\",\"type\":\"output\"}],\"Top\":[]}"
  Ref1 : PMIOPort  Side=Left
  Ref2 : PMIOPort  Port=2  Side=Right
  PLoss : Outport
  wires:
  PS-Simulink Converter1/1 -> Product/1
  PS-Simulink Converter/1 -> Subtract/1
  Product/1 -> Subtract/2
  Constant/1 -> Product/2
  Subtract/1 -> PLoss/1
  connections:
  Thermodynamic Properties Sensor (TL)/LConn1 -- Pressure & Temperature Sensor (TL)/RConn1 -- Ref2/RConn1
  PS-Simulink Converter/LConn1 -- Pressure & Temperature Sensor (TL)/RConn2
  Thermodynamic Properties Sensor (TL)/RConn2 -- PS-Simulink Converter1/LConn1
  Pressure & Temperature Sensor (TL)/LConn1 -- Ref1/RConn1

== system MSDRPrimaryLoop_LoadFollow/pipePumpToPHX/Subsystem ==
  note: Dh
  note: Dh
  note: Dh
  GasInRef : Inport
  2PModification : Subsystem  ReferencedSubsystem=TwoPhaseModification
      settings: PortSchema="{\"entries\":[{\"content\":{\"sides\":[{\"content\":{\"connectorIds\":[\"LConn1\"]},\"type\":\"ConnectorPlacement.EquallySpacedRectSide\",\"uuid\":\"7546b4b7-b669-49c8-8f27-f696391ea3ad\"},{\"content\":{\"connectorIds\":[\"RConn1\"],\"side\":\"RIGHT\"},\"type\":\"ConnectorPlacement.EquallySpacedRectSide\",\"uuid\":\"0e6176f2-177c-4327-bcfa-9a190fe9083f\"},{\"content\":{\"connectorIds\":[\"LConn2\"],\"side\":\"TOP\"},\"type\":\"ConnectorPlacement.EquallySpacedRectSide\",\"uuid\":\"16faf74c-4635-4009-a5b3-33dd03b625c6\"},{\"content\":{\"connectorIds\":[\"RConn2\",\"In1\"],\"side\":\"BOTTOM\"},\"type\":\"ConnectorPlacement.EquallySpacedRectSide\",\"uuid\":\"2081d73b-bb08-4ad9-b5c8-e48a4e9c4e20\"}]},\"type\":\"ConnectorPlacement.EquallySpacedConnector\",\"uuid\":\"243e4075-206b-4747-a8bc-b8f10d9a577f\"}],\"packageUris\":[\"http://schema.mathworks.com/mf0/Connector/R2020b\"],\"version\":\"1.0\"}"
  PS Abs : fl_lib/Physical Signals/Nonlinear Operators/PS Abs
      settings: SourceProductBaseCode=SS  InternalSimscapePortConfiguration="{\"Bottom\":[],\"Left\":[{\"id\":\"I\",\"label\":\"\",\"type\":\"input\"}],\"Right\":[{\"id\":\"O\",\"label\":\"\",\"type\":\"output\"}],\"Top\":[]}"
  Pipe (TL) : SimscapeFluids_lib/Thermal Liquid/Pipes & Fittings/Pipe (TL)  dynamic_compressibility=simscape.enum.onoff.on  inertia=simscape.enum.onoff.on  num_segments=1  pipe_length=Length m  area=Area m^2  Dh=0.1128 m  wall_spec=fluids.thermal_liquid.pipes_fittings.enum.wall_spec.rigid  Dh_rigid=Dh m  wall_compliance=1.2e-6 m/MPa  wall_time_constant=0.01 s  elevation_spec=foundation.enum.constant_variable.constant  elevation_gain=Elevation m  g=9.82 m/s^2  pressure_loss_spec=fluids.thermal_liquid.pipes_fittings.enum.PressureLossSpec.Haaland  length_add=1 m  roughness=15e-6 m  Re_friction_TLU=[400, 1000, 1500, 3000, 4000, 6000, 10000, 20000, 40000, 60000, 100000, 100000000]  friction_factor_TLU=[.264, .112, .071, .0417, .0387, .0268, .025, .0232, .0226, .022, .0214, .0214]  shape_factor=64  Re_lam=2000  Re_tur=4000  mdot_nominal=[.1, 1] kg/s  p_diff_nominal=[.001, .01] MPa  mdot_threshold=1e-6 kg/s  heat_transfer_spec=fluids.thermal_liquid.pipes_fittings.enum.HeatTransferSpec.Gnielinski  mdot_nominal_heat=[.1, 1] kg/s  T_in_nominal=[293.15, 293.15] K  T_out_nominal=[300, 300] K  p_in_nominal_heat=[.101325, .101325] MPa  T_wall_nominal=[303.15, 303.15] K  a_coeff=0.023  b_Re_power=0.8  c_Pr_power=0.4  Nu_lam=3.66  Re_Colburn_TLU=[100, 150, 1000]  Colburn_factor_TLU=[.019, .013, .002]  Re_Nu_TLU=[100, 150, 1000]  Pr_Nu_TLU=[1, 10]  Nu_TLU=[3.72, 4.21; 3.75, 4.44; 4.21, 7.15]  T0_vec=T0 K  p0_vec=P0 Pa  mdot0=0.1 kg/s
      settings: SourceProductBaseCode=SH  LogSimulationData=on
  Volumetric Flow Rate Sensor (TL) : fl_lib/Thermal Liquid/Sensors/Volumetric Flow Rate Sensor (TL)
      settings: SourceProductBaseCode=SS  InternalSimscapePortConfiguration="{\"Bottom\":[],\"Left\":[{\"id\":\"A\",\"label\":\"A\",\"type\":\"foundation.thermal_liquid.thermal_liquid\"}],\"Right\":[{\"id\":\"B\",\"label\":\"B\",\"type\":\"foundation.thermal_liquid.thermal_liquid\"},{\"id\":\"V\",\"label\":\"V\",\"type\":\"output\"}],\"Top\":[]}"
  Inlet : PMIOPort  Side=Left
  Outlet : PMIOPort  Port=2  Side=Right
  VolumeRate : PMIOPort  Port=3  Side=Right
  wires:
  GasInRef/1 -> 2PModification/1
  connections:
  Volumetric Flow Rate Sensor (TL)/RConn1 -- Pipe (TL)/LConn1
  Inlet/RConn1 -- 2PModification/LConn2 -- Volumetric Flow Rate Sensor (TL)/LConn1
  Pipe (TL)/RConn1 -- 2PModification/RConn2 -- 2PModification/LConn1
  Volumetric Flow Rate Sensor (TL)/RConn2 -- PS Abs/LConn1
  PS Abs/RConn1 -- VolumeRate/RConn1
  2PModification/RConn1 -- Outlet/RConn1

== system MSDRPrimaryLoop_LoadFollow/pipePumpToPHX/XenonCalc ==
  XeIn : Inport  OutDataTypeStr=double  Unit=kg/s
  PLoss : Inport  Port=2
  GasRef : Inport  Port=3
  Absolute Reference (TL) : fl_lib/Thermal Liquid/Elements/Absolute Reference (TL)
      settings: SourceProductBaseCode=SS
  Demux : Demux  Outputs=2
  Gas : Subsystem
      settings: PortSchema="{\"entries\":[{\"content\":{\"sides\":[{\"content\":{\"connectorIds\":[\"In1\"]},\"type\":\"ConnectorPlacement.EquallySpacedRectSide\",\"uuid\":\"9457d014-8c8c-4ede-953a-dad1b8fcff2e\"},{\"content\":{\"connectorIds\":[\"Out1\"],\"side\":\"RIGHT\"},\"type\":\"ConnectorPlacement.EquallySpacedRectSide\",\"uuid\":\"6b13e550-1648-4662-a58b-f6f49b8dfc45\"},{\"content\":{\"connectorIds\":[\"Out2\",\"In2\"],\"side\":\"TOP\"},\"type\":\"ConnectorPlacement.EquallySpacedRectSide\",\"uuid\":\"73a4211d-b4c2-4f72-9c26-6ee46c1777bd\"},{\"content\":{\"connectorIds\":[\"In3\",\"In4\"],\"side\":\"BOTTOM\"},\"type\":\"ConnectorPlacement.EquallySpacedRectSide\",\"uuid\":\"ca62b0cd-46c8-418f-9a8b-9558726bf444\"}]},\"type\":\"ConnectorPlacement.EquallySpacedConnector\",\"uuid\":\"020f2da1-56fe-4a8a-8a2d-2f75d9123e14\"}],\"packageUris\":[\"http://schema.mathworks.com/mf0/Connector/R2020b\"],\"version\":\"1.0\"}"
  InterphaseTranfser : Subsystem
      settings: PortSchema="{\"entries\":[{\"content\":{\"sides\":[{\"content\":{\"connectorIds\":[\"In1\",\"In2\",\"In3\"]},\"type\":\"ConnectorPlacement.EquallySpacedRectSide\",\"uuid\":\"d6303689-138e-451a-a3c3-60d601b4795c\"},{\"content\":{\"connectorIds\":[\"In5\",\"Out1\"],\"side\":\"RIGHT\"},\"type\":\"ConnectorPlacement.EquallySpacedRectSide\",\"uuid\":\"e99266db-1ad9-4248-a3a9-dc80edd4cbf2\"},{\"content\":{\"connectorIds\":[\"LConn1\"],\"side\":\"TOP\"},\"type\":\"ConnectorPlacement.EquallySpacedRectSide\",\"uuid\":\"07679a3e-e535-452f-8d16-cac9376cf8bb\"},{\"content\":{\"connectorIds\":[\"In4\"],\"side\":\"BOTTOM\"},\"type\":\"ConnectorPlacement.EquallySpacedRectSide\",\"uuid\":\"cd334689-6a33-4cbf-8721-40055306f60f\"}]},\"type\":\"ConnectorPlacement.EquallySpacedConnector\",\"uuid\":\"2a8870ca-366d-4312-85a0-e0a2095078d0\"}],\"packageUris\":[\"http://schema.mathworks.com/mf0/Connector/R2020b\"],\"version\":\"1.0\"}"
  Mux : Mux  Inputs=2
  PS Abs : fl_lib/Physical Signals/Nonlinear Operators/PS Abs
      settings: SourceProductBaseCode=SS  InternalSimscapePortConfiguration="{\"Bottom\":[],\"Left\":[{\"id\":\"I\",\"label\":\"\",\"type\":\"input\"}],\"Right\":[{\"id\":\"O\",\"label\":\"\",\"type\":\"output\"}],\"Top\":[]}"
  PS-Simulink Converter : nesl_utility/PS-Simulink Converter  PhysicalDomain=network_engine_domain  SubClassName=ps_output  LeftPortType=input  RightPortType=output  PseudoPeriodic=off  Frequencies=[]  Unit=inherit  AffineConversion=off
      settings: SourceProductBaseCode=PW,SS
  PS-Simulink Converter1 : nesl_utility/PS-Simulink Converter  PhysicalDomain=network_engine_domain  SubClassName=ps_output  LeftPortType=input  RightPortType=output  PseudoPeriodic=off  Frequencies=[]  Unit=inherit  AffineConversion=off
      settings: SourceProductBaseCode=PW,SS
  Pressure & Temperature Sensor (TL) : fl_lib/Thermal Liquid/Sensors/Pressure & Temperature Sensor (TL)
      settings: SourceProductBaseCode=SS  InternalSimscapePortConfiguration="{\"Bottom\":[],\"Left\":[{\"id\":\"A\",\"label\":\"A\",\"type\":\"foundation.thermal_liquid.thermal_liquid\"}],\"Right\":[{\"id\":\"B\",\"label\":\"B\",\"type\":\"foundation.thermal_liquid.thermal_liquid\"},{\"id\":\"P\",\"label\":\"P\",\"type\":\"output\"},{\"id\":\"T\",\"label\":\"T\",\"type\":\"output\"}],\"Top\":[]}"
  Salt : Subsystem
      settings: PortSchema="{\"entries\":[{\"content\":{\"sides\":[{\"content\":{\"connectorIds\":[\"In1\",\"In2\",\"In3\"]},\"type\":\"ConnectorPlacement.EquallySpacedRectSide\",\"uuid\":\"9457d014-8c8c-4ede-953a-dad1b8fcff2e\"},{\"content\":{\"connectorIds\":[\"Out1\"],\"side\":\"RIGHT\"},\"type\":\"ConnectorPlacement.EquallySpacedRectSide\",\"uuid\":\"6b13e550-1648-4662-a58b-f6f49b8dfc45\"},{\"content\":{\"connectorIds\":[\"In4\",\"In5\"],\"side\":\"TOP\"},\"type\":\"ConnectorPlacement.EquallySpacedRectSide\",\"uuid\":\"73a4211d-b4c2-4f72-9c26-6ee46c1777bd\"},{\"content\":{\"connectorIds\":[\"Out2\",\"In6\"],\"side\":\"BOTTOM\"},\"type\":\"ConnectorPlacement.EquallySpacedRectSide\",\"uuid\":\"ca62b0cd-46c8-418f-9a8b-9558726bf444\"}]},\"type\":\"ConnectorPlacement.EquallySpacedConnector\",\"uuid\":\"020f2da1-56fe-4a8a-8a2d-2f75d9123e14\"}],\"packageUris\":[\"http://schema.mathworks.com/mf0/Connector/R2020b\"],\"version\":\"1.0\"}"
  Volumetric Flow Rate Sensor (TL) : fl_lib/Thermal Liquid/Sensors/Volumetric Flow Rate Sensor (TL)
      settings: SourceProductBaseCode=SS  InternalSimscapePortConfiguration="{\"Bottom\":[],\"Left\":[{\"id\":\"A\",\"label\":\"A\",\"type\":\"foundation.thermal_liquid.thermal_liquid\"}],\"Right\":[{\"id\":\"B\",\"label\":\"B\",\"type\":\"foundation.thermal_liquid.thermal_liquid\"},{\"id\":\"V\",\"label\":\"V\",\"type\":\"output\"}],\"Top\":[]}"
  Inlet : PMIOPort  Side=Left
  Outlet : PMIOPort  Port=2  Side=Right
  XeOut : Outport
  wires:
  XeIn/1 -> Demux/1
  PS-Simulink Converter/1 -> InterphaseTranfser/5(VolumeRate), Gas/4(VolumeRate), Salt/5(VolumeRate)
  GasRef/1 -> Gas/3(GasRef), InterphaseTranfser/2(GasRef), Salt/4(GasRef)
  Demux/1 -> Salt/1(XeLIn)
  [IodineSNDensity] -> Salt/2(IodineSNumberDensity)
  Demux/2 -> Gas/1(XeGIn)
  Salt/1(XeLOut) -> Mux/1
  Gas/1(XeGOut) -> Mux/2
  Mux/1 -> XeOut/1
  Salt/2(GxSalt) -> InterphaseTranfser/1(GxSalt)
  Gas/2(GxGas) -> InterphaseTranfser/3(GxGas)
  InterphaseTranfser/1(TranfserRate) -> Salt/6(Interphase), Gas/2(Interphase)
  PS-Simulink Converter1/1 -> Salt/3(T_f_ave)
  PLoss/1 -> InterphaseTranfser/4(PLoss)
  connections:
  Outlet/RConn1 -- Volumetric Flow Rate Sensor (TL)/RConn1 -- InterphaseTranfser/LConn1
  Volumetric Flow Rate Sensor (TL)/LConn1 -- Pressure & Temperature Sensor (TL)/LConn1 -- Inlet/RConn1
  Volumetric Flow Rate Sensor (TL)/RConn2 -- PS Abs/LConn1
  PS Abs/RConn1 -- PS-Simulink Converter/LConn1
  Pressure & Temperature Sensor (TL)/RConn1 -- Absolute Reference (TL)/LConn1
  Pressure & Temperature Sensor (TL)/RConn3 -- PS-Simulink Converter1/LConn1

== system MSDRPrimaryLoop_LoadFollow/pipeReactorToPump/GasCalc ==
  GasIn : Inport
  Add : Sum  Inputs=+-
  GasExpansion : Subsystem  ReferencedSubsystem=GasExpansion
      settings: PortSchema="{\"entries\":[{\"content\":{\"sides\":[{\"content\":{\"connectorIds\":[\"LConn1\",\"In1\"]},\"type\":\"ConnectorPlacement.EquallySpacedRectSide\",\"uuid\":\"50c89675-cb8a-4964-af62-cb2014507b1d\"},{\"content\":{\"connectorIds\":[\"RConn1\",\"Out1\"],\"side\":\"RIGHT\"},\"type\":\"ConnectorPlacement.EquallySpacedRectSide\",\"uuid\":\"6b3adc78-0be5-4682-9da0-6fd41ffc4e71\"},{\"content\":{\"connectorIds\":[],\"side\":\"TOP\"},\"type\":\"ConnectorPlacement.EquallySpacedRectSide\",\"uuid\":\"5158b46f-a496-48e4-90d6-6c6dcc9e237b\"}]},\"type\":\"ConnectorPlacement.EquallySpacedConnector\",\"uuid\":\"7ff0188e-dc19-44a0-a8cf-bde33949414f\"}],\"packageUris\":[\"http://schema.mathworks.com/mf0/Connector/R2020b\"],\"version\":\"1.0\"}"
  Integrator : Integrator
  PS-Simulink Converter : nesl_utility/PS-Simulink Converter  PhysicalDomain=network_engine_domain  SubClassName=ps_output  LeftPortType=input  RightPortType=output  PseudoPeriodic=off  Frequencies=[]  Unit=inherit  AffineConversion=off
      settings: SourceProductBaseCode=PW,SS
  Product : Product
  VolumeToVoid : Gain  Gain=1/Volume
  Ref1 : PMIOPort  Side=Left
  VolumeRate : PMIOPort  Port=2  Side=Left
  Ref2 : PMIOPort  Port=3  Side=Left
  GasOut : Outport
  wires:
  VolumeToVoid/1 -> GasExpansion/1, Add/2
  Integrator/1 -> VolumeToVoid/1
  GasIn/1 -> Add/1
  Add/1 -> Product/1
  Product/1 -> Integrator/1
  PS-Simulink Converter/1 -> Product/2
  GasExpansion/1 -> GasOut/1
  connections:
  PS-Simulink Converter/LConn1 -- VolumeRate/RConn1
  GasExpansion/LConn1 -- Ref1/RConn1
  GasExpansion/RConn1 -- Ref2/RConn1
